simulink model "my_exp1_hover"  (R2022b)
settings: Solver=VariableStepAuto  StartTime=0.0  StopTime=10.0  RelTol=1e-3
values from neighbouring files (symbols this model uses):
  f1234tofm = [1 1 1 1 ... (first row only)    [my_exp1.m]
  fmtof1234 = inv(f1234tofm)    [my_exp1.m]
  g = 9.8    [my_exp1.m]
  Ixx = 0.003    [my_exp1.m]
  Iyy = 0.003    [my_exp1.m]
  Izz = 0.005    [my_exp1.m]
  k_F = 1.9e-8    (= 1.9e-08)    [my_exp1.m]
  k_m = 100    [my_exp1.m]
  m = 0.8    [my_exp1.m]
  maxz = 25000    [my_exp1.m]
  minz = 10000    [my_exp1.m]
libraries: shared6dof x1
settings Model: Creator=zzy  LastModifiedBy=zzy

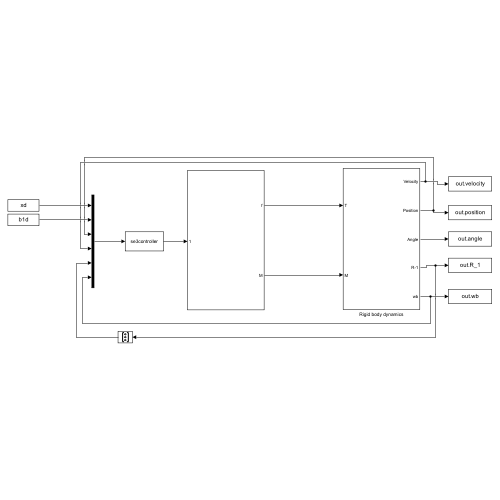
[thumbnail: Simulink's stored preview of the top-level diagram]
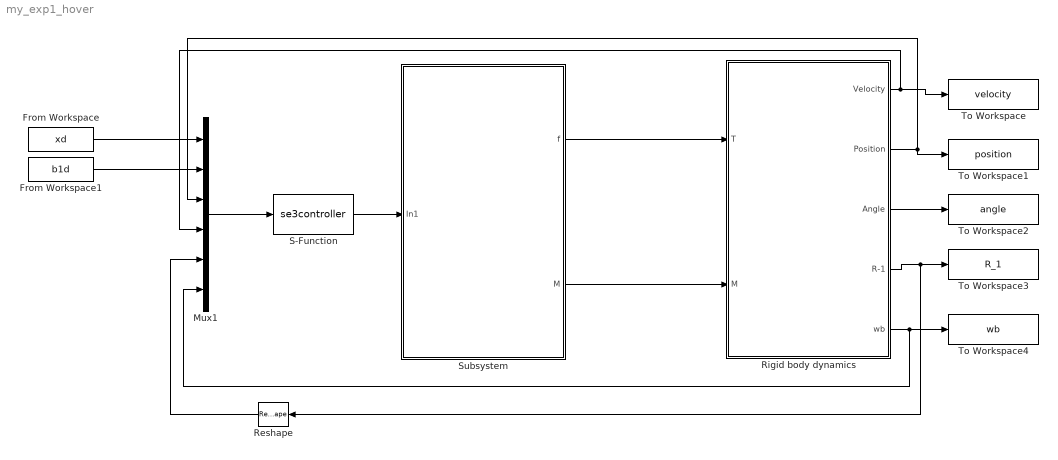
== system my_exp1_hover ==
  From Workspace : FromWorkspace  VariableName=xd
  From Workspace1 : FromWorkspace  VariableName=b1d
  Mux1 : Mux  Inputs=6
  Reshape : Reshape  OutputDimensionality=Column vector (2-D)
  Rigid body dynamics : Subsystem
  S-Function : S-Function  FunctionName=se3controller  SFunctionDeploymentMode=off  EnableBusSupport=off
  Subsystem : Subsystem
  To Workspace : ToWorkspace  VariableName=velocity  SampleTime=-1
      settings: Save2DSignal=2-D array (concatenate along first dimension)
  To Workspace1 : ToWorkspace  VariableName=position  SampleTime=-1
      settings: Save2DSignal=2-D array (concatenate along first dimension)
  To Workspace2 : ToWorkspace  VariableName=angle  SampleTime=-1
      settings: Save2DSignal=2-D array (concatenate along first dimension)
  To Workspace3 : ToWorkspace  VariableName=R_1  SampleTime=-1
      settings: Save2DSignal=2-D array (concatenate along first dimension)
  To Workspace4 : ToWorkspace  VariableName=wb  SampleTime=-1
      settings: Save2DSignal=2-D array (concatenate along first dimension)
  wires:
  Rigid body dynamics/2(Position) -> To Workspace1/1, Mux1/3
  Rigid body dynamics/1(Velocity) -> Mux1/4, To Workspace/1
  Rigid body dynamics/3(Angle) -> To Workspace2/1
  Rigid body dynamics/4(R-1) -> Reshape/1, To Workspace3/1
  Rigid body dynamics/5(wb) -> Mux1/6, To Workspace4/1
  From Workspace/1 -> Mux1/1
  From Workspace1/1 -> Mux1/2
  Mux1/1 -> S-Function/1
  Reshape/1 -> Mux1/5
  S-Function/1 -> Subsystem/1(In1)
  Subsystem/1(f) -> Rigid body dynamics/1(T)
  Subsystem/2(M) -> Rigid body dynamics/2(M)

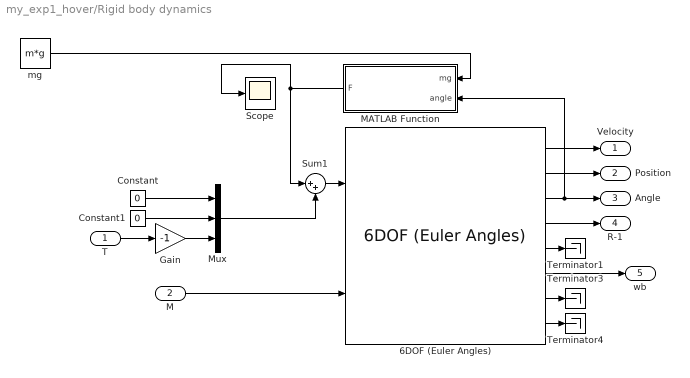
== system my_exp1_hover/Rigid body dynamics ==
  T : Inport
  M : Inport  Port=2
  6DOF (Euler Angles) : shared6dof/6DOF (Euler Angles)  units=Metric (MKS)  mtype=Fixed  rep=Quaternion  xme_0=[0 0 0]  Vm_0=[0 0 0]  eul_0=[0 0 0]  pm_0=[0 0 0]  mass_0=m  mass_e=0.5  mass_f=2.0  inertia=[Ixx,0,0; 0,Iyy,0; 0,0,Izz]  inertia_e=eye(3)  inertia_f=2*eye(3)  k_quat=1.0  vre_flag=on  abi_flag=off  aMode=0  xme_statename=''  Vm_statename=''  eul_statename=''  quat_statename=''  pm_statename=''  mass_statename=''
  Constant : Constant  Value=0
  Constant1 : Constant  Value=0
  Gain : Gain  Gain=-1
  MATLAB Function : MATLAB Function  TreatAsAtomicUnit=on
  Mux : Mux  Inputs=3
  Scope : Scope
  Sum1 : Sum  Inputs=|++
  Terminator1 : Terminator
  Terminator3 : Terminator
  Terminator4 : Terminator
  mg : Constant  Value=m*g
  Velocity : Outport
  Position : Outport  Port=2
  Angle : Outport  Port=3
  R-1 : Outport  Port=4
  wb : Outport  Port=5
  wires:
  6DOF (Euler Angles)/1 -> Velocity/1
  6DOF (Euler Angles)/3 -> MATLAB Function/2(angle), Angle/1
  6DOF (Euler Angles)/2 -> Position/1
  M/1 -> 6DOF (Euler Angles)/2
  Sum1/1 -> 6DOF (Euler Angles)/1
  6DOF (Euler Angles)/4 -> R-1/1
  6DOF (Euler Angles)/6 -> wb/1
  6DOF (Euler Angles)/7 -> Terminator3/1
  6DOF (Euler Angles)/8 -> Terminator4/1
  mg/1 -> MATLAB Function/1(mg)
  MATLAB Function/1(F) -> Sum1/1, Scope/1
  6DOF (Euler Angles)/5 -> Terminator1/1
  T/1 -> Gain/1
  Constant/1 -> Mux/1
  Constant1/1 -> Mux/2
  Mux/1 -> Sum1/2
  Gain/1 -> Mux/3

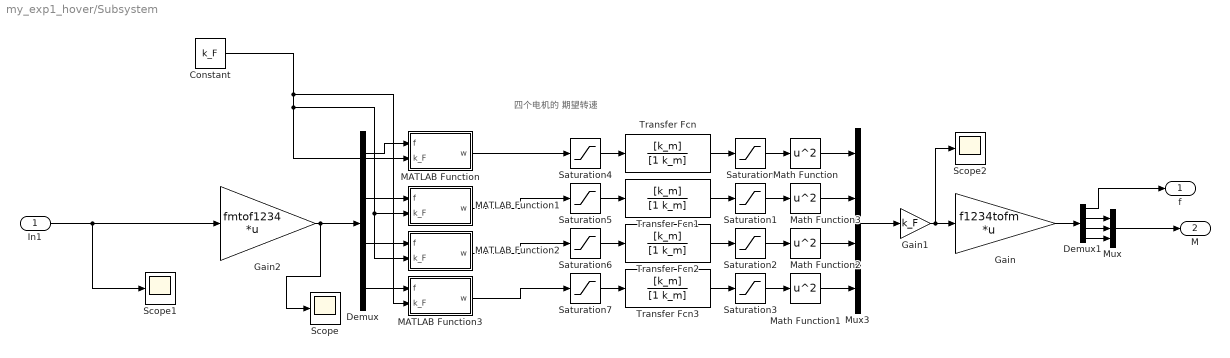
== system my_exp1_hover/Subsystem ==
  note: 四个电机的
      | 期望转速
  In1 : Inport
  Constant : Constant  Value=k_F
  Demux : Demux
  Demux1 : Demux
  Gain : Gain  Gain=f1234tofm  Multiplication=Matrix(K*u) (u vector)
  Gain1 : Gain  Gain=k_F
  Gain2 : Gain  Gain=fmtof1234  Multiplication=Matrix(K*u) (u vector)
  MATLAB Function : MATLAB Function  TreatAsAtomicUnit=on
  MATLAB Function1 : MATLAB Function  TreatAsAtomicUnit=on
  MATLAB Function2 : MATLAB Function  TreatAsAtomicUnit=on
  MATLAB Function3 : MATLAB Function  TreatAsAtomicUnit=on
  Math Function{,1..3} (4 alike) : Math  Operator=square
  Mux : Mux  Inputs=3
  Mux3 : Mux
  Saturation{,1..7} (8 alike) : Saturate  UpperLimit=maxz  LowerLimit=minz
  Scope : Scope
  Scope1 : Scope
  Scope2 : Scope
  Transfer Fcn{,1..3} (4 alike) : TransferFcn  Numerator=[k_m]  Denominator=[1 k_m]
  f : Outport
  M : Outport  Port=2
  wires:
  MATLAB Function/1(w) -> Saturation4/1
  Demux/3 -> MATLAB Function2/1(f)
  Saturation5/1 -> Transfer Fcn1/1
  Saturation1/1 -> Math Function3/1
  Math Function/1 -> Mux3/1
  Saturation2/1 -> Math Function2/1
  Math Function2/1 -> Mux3/3
  Math Function1/1 -> Mux3/4
  In1/1 -> Scope1/1, Gain2/1
  Demux/2 -> MATLAB Function1/1(f)
  Saturation3/1 -> Math Function1/1
  Transfer Fcn2/1 -> Saturation2/1
  MATLAB Function3/1(w) -> Saturation7/1
  Saturation/1 -> Math Function/1
  Demux/4 -> MATLAB Function3/1(f)
  Demux/1 -> MATLAB Function/1(f)
  Mux3/1 -> Gain1/1
  MATLAB Function2/1(w) -> Saturation6/1
  MATLAB Function1/1(w) -> Saturation5/1
  Gain2/1 -> Scope/1, Demux/1
  Saturation7/1 -> Transfer Fcn3/1
  Saturation4/1 -> Transfer Fcn/1
  Transfer Fcn3/1 -> Saturation3/1
  Saturation6/1 -> Transfer Fcn2/1
  Transfer Fcn1/1 -> Saturation1/1
  Math Function3/1 -> Mux3/2
  Transfer Fcn/1 -> Saturation/1
  Gain/1 -> Demux1/1
  Demux1/2 -> Mux/1
  Demux1/3 -> Mux/2
  Demux1/4 -> Mux/3
  Demux1/1 -> f/1
  Mux/1 -> M/1
  Constant/1 -> MATLAB Function3/2(k_F), MATLAB Function2/2(k_F), MATLAB Function1/2(k_F), MATLAB Function/2(k_F)
  Gain1/1 -> Scope2/1, Gain/1

== matlab function my_exp1_hover/Rigid body dynamics/MATLAB Function ==
  data: mg input; angle input; F output
function F = mg_w2b(mg, angle)
phi = angle(1);
theta = angle(2);
F = [-sin(theta);cos(theta)*sin(phi);cos(phi)*cos(theta)] * mg;

== matlab function my_exp1_hover/Subsystem/MATLAB Function1 ==
  data: f input; w output; k_F input
function w = f2w(f,k_F)
if f>0
    w=sqrt(f/k_F);
else
    w=0;
end

== matlab function my_exp1_hover/Subsystem/MATLAB Function2 ==
  data: f input; w output; k_F input
function w = f2w(f,k_F)
if f>0
    w=sqrt(f/k_F);
else
    w=0;
end

== matlab function my_exp1_hover/Subsystem/MATLAB Function3 ==
  data: f input; w output; k_F input
function w = f2w(f,k_F)
if f>0
    w=sqrt(f/k_F);
else
    w=0;
end

== matlab function my_exp1_hover/Subsystem/MATLAB Function ==
  data: f input; w output; k_F input
function w = f2w(f,k_F)
if f>0
    w=sqrt(f/k_F);
else
    w=0;
end
